simulink model "feedbackLinearizationMambo"  (R2021a)
settings: Solver=VariableStepAuto  StartTime=0.0  StopTime=10  FixedStep=4e-3  RelTol=1e-12
InitFcn:
  | init
values from neighbouring files (symbols this model uses):
  a = 4.7200e-08*13840.8    (= 0.00065328576)    [init.m]
  c = 1.1393e-10*13840.8    (= 1.576882344e-06)    [init.m]
  g = 9.31    [init.m]
  isMambo = true    [init.m]
  J = [Jx;Jy;Jz]    [init.m]
  Jx = 5.82857e-5    (= 5.82857e-05)    [init.m]
  Jy = 7.169148e-5    (= 7.169148e-05)    [init.m]
  Jz = 1e-4    (= 0.0001)    [init.m]
  Ki = [0.1 0.6 0.1]*0    [init.m]
  Kp = [0.6 0.7 1]*50    [init.m]
  Kw = [0.08 0.1 0.2]*100    [init.m]
  l = 0.0624*2    (= 0.1248)    [init.m]
  m = 0.063    [init.m]
  posNED = [57 95 -0.046]    [init.m]
  sigma = [l*a/Jx l*a/Jy l*a/Jz a/m]    [init.m]
  T = 0.0050    (= 0.005)    [init.m]
undefined symbols (not defined in the file or in its folder): DiscIntNeverNeededParam, Earth, init, rho, Vehicle, WGS84
libraries: pid_lib x14, sharedtransform x6, simulink x2, shared6dof x1, aerolibasang x1, aerolibtransform2 x1, vrlib x1
(part 2 of 2)

== system feedbackLinearizationMambo/Controller2/PD Mambo ==
  e : Inport
  Demux : Demux
  Discrete PID Controller : pid_lib/PID Controller  Controller=PD  Form=Parallel  TimeDomain=Discrete-time  UseExternalTs=off  SampleTime=T  IntegratorMethod=Forward Euler  FilterMethod=Forward Euler  ControllerParametersSource=internal  P=0.625617124169113  I=Ki  D=7.14769061437549  UseFilter=on  N=296.310341187165  TunerSelectOption=Transfer Function Based (PID Tuner App)  InitialConditionSource=internal  InitialConditionForIntegrator=0  InitialConditionForFilter=0  DifferentiatorICPrevScaledInput=0  ExternalReset=none  TrackingMode=off  Kt=1  LimitOutput=off  SatLimitsSource=internal  UpperSaturationLimit=inf  LowerSaturationLimit=-inf  LinearizeAsGain=off  AntiWindupMode=none  Kb=1  POutMin=[]  POutMax=[]  IOutMin=[]  IOutMax=[]  DOutMin=[]  DOutMax=[]  NOutMin=[]  NOutMax=[]  SumOutMin=[]  SumOutMax=[]  SaturationOutMin=[]  SaturationOutMax=[]  PParamMin=[]  PParamMax=[]  IParamMin=[]  IParamMax=[]  DParamMin=[]  DParamMax=[]  NParamMin=[]  NParamMax=[]  KbParamMin=[]  KbParamMax=[]  KtParamMin=[]  KtParamMax=[]  KbOutMin=[]  KbOutMax=[]  KtOutMin=[]  KtOutMax=[]  IntegratorOutMin=[]  IntegratorOutMax=[]  FilterOutMin=[]  FilterOutMax=[]  SumI1OutMin=[]  SumI1OutMax=[]  SumI2OutMin=[]  SumI2OutMax=[]  SumI3OutMin=[]  SumI3OutMax=[]  SumI4OutMin=[]  SumI4OutMax=[]  SumDOutMin=[]  SumDOutMax=[]  DifferentiatorOutMin=[]  DifferentiatorOutMax=[]  FilterDiffOutCoefMin=[]  FilterDiffOutCoefMax=[]  ReciprocalOutMin=[]  ReciprocalOutMax=[]  SumDenOutMin=[]  SumDenOutMax=[]  SumNumOutMin=[]  SumNumOutMax=[]  DivideOutMin=[]  DivideOutMax=[]  UdiffTsProdOutMin=[]  UdiffTsProdOutMax=[]  NTsProdOutMin=[]  NTsProdOutMax=[]  UintegralTsProdOutMin=[]  UintegralTsProdOutMax=[]  UngainTsProdOutMin=[]  UngainTsProdOutMax=[]  IntegratorContinuousStateAttributes=''  IntegratorStateMustResolveToSignalObject=off  IntegratorRTWStateStorageClass=Auto  FilterContinuousStateAttributes=''  FilterStateMustResolveToSignalObject=off  FilterRTWStateStorageClass=Auto  ParallelPVariant=InternalParameters  IdealPVariant=Disabled  IVariant=Disabled  DVariant=InternalParameters  IntegratorVariant=Disabled  SatVariant=Disabled  AWVariant=Disabled  PCopyVariant=Disabled  TRVariant=Disabled  FdbkBlocksVariant=Forward  IdealPFdbkVariant=Disabled  SatFdbkVariant=Disabled  DerivativeFilterVariant=ForwardEulerFilter  NVariant=InternalParameters  NCopyVariant=Disabled  FilterICVariant=InternalICsFilter  IntegratorICVariant=Disabled  ExternalResetVariant=Disabled  TRSumVariant=Passthrough  SumFdbkVariant=Disabled  SumVariant=Sum_PD  TsampFilterVariant=InternalTs  TsampNgainVariant=Passthrough  TsampIntegralVariant=Disabled_SignalSpec  ExternalSaturationOutDataTypeStr=Inherit: Same as second input
  Discrete PID Controller1 : pid_lib/PID Controller  Controller=PD  Form=Parallel  TimeDomain=Discrete-time  UseExternalTs=off  SampleTime=T  IntegratorMethod=Forward Euler  FilterMethod=Forward Euler  ControllerParametersSource=internal  P=0.769509803348267  I=Ki  D=8.79166791728825  UseFilter=on  N=296.310341187165  TunerSelectOption=Transfer Function Based (PID Tuner App)  InitialConditionSource=internal  InitialConditionForIntegrator=0  InitialConditionForFilter=0  DifferentiatorICPrevScaledInput=0  ExternalReset=none  TrackingMode=off  Kt=1  LimitOutput=off  SatLimitsSource=internal  UpperSaturationLimit=inf  LowerSaturationLimit=-inf  LinearizeAsGain=off  AntiWindupMode=none  Kb=1  POutMin=[]  POutMax=[]  IOutMin=[]  IOutMax=[]  DOutMin=[]  DOutMax=[]  NOutMin=[]  NOutMax=[]  SumOutMin=[]  SumOutMax=[]  SaturationOutMin=[]  SaturationOutMax=[]  PParamMin=[]  PParamMax=[]  IParamMin=[]  IParamMax=[]  DParamMin=[]  DParamMax=[]  NParamMin=[]  NParamMax=[]  KbParamMin=[]  KbParamMax=[]  KtParamMin=[]  KtParamMax=[]  KbOutMin=[]  KbOutMax=[]  KtOutMin=[]  KtOutMax=[]  IntegratorOutMin=[]  IntegratorOutMax=[]  FilterOutMin=[]  FilterOutMax=[]  SumI1OutMin=[]  SumI1OutMax=[]  SumI2OutMin=[]  SumI2OutMax=[]  SumI3OutMin=[]  SumI3OutMax=[]  SumI4OutMin=[]  SumI4OutMax=[]  SumDOutMin=[]  SumDOutMax=[]  DifferentiatorOutMin=[]  DifferentiatorOutMax=[]  FilterDiffOutCoefMin=[]  FilterDiffOutCoefMax=[]  ReciprocalOutMin=[]  ReciprocalOutMax=[]  SumDenOutMin=[]  SumDenOutMax=[]  SumNumOutMin=[]  SumNumOutMax=[]  DivideOutMin=[]  DivideOutMax=[]  UdiffTsProdOutMin=[]  UdiffTsProdOutMax=[]  NTsProdOutMin=[]  NTsProdOutMax=[]  UintegralTsProdOutMin=[]  UintegralTsProdOutMax=[]  UngainTsProdOutMin=[]  UngainTsProdOutMax=[]  IntegratorContinuousStateAttributes=''  IntegratorStateMustResolveToSignalObject=off  IntegratorRTWStateStorageClass=Auto  FilterContinuousStateAttributes=''  FilterStateMustResolveToSignalObject=off  FilterRTWStateStorageClass=Auto  ParallelPVariant=InternalParameters  IdealPVariant=Disabled  IVariant=Disabled  DVariant=InternalParameters  IntegratorVariant=Disabled  SatVariant=Disabled  AWVariant=Disabled  PCopyVariant=Disabled  TRVariant=Disabled  FdbkBlocksVariant=Forward  IdealPFdbkVariant=Disabled  SatFdbkVariant=Disabled  DerivativeFilterVariant=ForwardEulerFilter  NVariant=InternalParameters  NCopyVariant=Disabled  FilterICVariant=InternalICsFilter  IntegratorICVariant=Disabled  ExternalResetVariant=Disabled  TRSumVariant=Passthrough  SumFdbkVariant=Disabled  SumVariant=Sum_PD  TsampFilterVariant=InternalTs  TsampNgainVariant=Passthrough  TsampIntegralVariant=Disabled_SignalSpec  ExternalSaturationOutDataTypeStr=Inherit: Same as second input
  Discrete PID Controller2 : pid_lib/PID Controller  Controller=PD  Form=Parallel  TimeDomain=Discrete-time  UseExternalTs=off  SampleTime=T  IntegratorMethod=Forward Euler  FilterMethod=Forward Euler  ControllerParametersSource=internal  P=130.980048513602  I=Ki  D=195.85931761802  UseFilter=on  N=189.861187655288  TunerSelectOption=Transfer Function Based (PID Tuner App)  InitialConditionSource=internal  InitialConditionForIntegrator=0  InitialConditionForFilter=0  DifferentiatorICPrevScaledInput=0  ExternalReset=none  TrackingMode=off  Kt=1  LimitOutput=off  SatLimitsSource=internal  UpperSaturationLimit=inf  LowerSaturationLimit=-inf  LinearizeAsGain=off  AntiWindupMode=none  Kb=1  POutMin=[]  POutMax=[]  IOutMin=[]  IOutMax=[]  DOutMin=[]  DOutMax=[]  NOutMin=[]  NOutMax=[]  SumOutMin=[]  SumOutMax=[]  SaturationOutMin=[]  SaturationOutMax=[]  PParamMin=[]  PParamMax=[]  IParamMin=[]  IParamMax=[]  DParamMin=[]  DParamMax=[]  NParamMin=[]  NParamMax=[]  KbParamMin=[]  KbParamMax=[]  KtParamMin=[]  KtParamMax=[]  KbOutMin=[]  KbOutMax=[]  KtOutMin=[]  KtOutMax=[]  IntegratorOutMin=[]  IntegratorOutMax=[]  FilterOutMin=[]  FilterOutMax=[]  SumI1OutMin=[]  SumI1OutMax=[]  SumI2OutMin=[]  SumI2OutMax=[]  SumI3OutMin=[]  SumI3OutMax=[]  SumI4OutMin=[]  SumI4OutMax=[]  SumDOutMin=[]  SumDOutMax=[]  DifferentiatorOutMin=[]  DifferentiatorOutMax=[]  FilterDiffOutCoefMin=[]  FilterDiffOutCoefMax=[]  ReciprocalOutMin=[]  ReciprocalOutMax=[]  SumDenOutMin=[]  SumDenOutMax=[]  SumNumOutMin=[]  SumNumOutMax=[]  DivideOutMin=[]  DivideOutMax=[]  UdiffTsProdOutMin=[]  UdiffTsProdOutMax=[]  NTsProdOutMin=[]  NTsProdOutMax=[]  UintegralTsProdOutMin=[]  UintegralTsProdOutMax=[]  UngainTsProdOutMin=[]  UngainTsProdOutMax=[]  IntegratorContinuousStateAttributes=''  IntegratorStateMustResolveToSignalObject=off  IntegratorRTWStateStorageClass=Auto  FilterContinuousStateAttributes=''  FilterStateMustResolveToSignalObject=off  FilterRTWStateStorageClass=Auto  ParallelPVariant=InternalParameters  IdealPVariant=Disabled  IVariant=Disabled  DVariant=InternalParameters  IntegratorVariant=Disabled  SatVariant=Disabled  AWVariant=Disabled  PCopyVariant=Disabled  TRVariant=Disabled  FdbkBlocksVariant=Forward  IdealPFdbkVariant=Disabled  SatFdbkVariant=Disabled  DerivativeFilterVariant=ForwardEulerFilter  NVariant=InternalParameters  NCopyVariant=Disabled  FilterICVariant=InternalICsFilter  IntegratorICVariant=Disabled  ExternalResetVariant=Disabled  TRSumVariant=Passthrough  SumFdbkVariant=Disabled  SumVariant=Sum_PD  TsampFilterVariant=InternalTs  TsampNgainVariant=Passthrough  TsampIntegralVariant=Disabled_SignalSpec  ExternalSaturationOutDataTypeStr=Inherit: Same as second input
  Discrete PID Controller3 : pid_lib/PID Controller  Controller=PD  Form=Parallel  TimeDomain=Discrete-time  UseExternalTs=off  SampleTime=T  IntegratorMethod=Forward Euler  FilterMethod=Forward Euler  ControllerParametersSource=internal  P=0.0348354109151771  I=Ki  D=1.99510127130573  UseFilter=on  N=145.233498095858  TunerSelectOption=Transfer Function Based (PID Tuner App)  InitialConditionSource=internal  InitialConditionForIntegrator=0  InitialConditionForFilter=0  DifferentiatorICPrevScaledInput=0  ExternalReset=none  TrackingMode=off  Kt=1  LimitOutput=off  SatLimitsSource=internal  UpperSaturationLimit=inf  LowerSaturationLimit=-inf  LinearizeAsGain=off  AntiWindupMode=none  Kb=1  POutMin=[]  POutMax=[]  IOutMin=[]  IOutMax=[]  DOutMin=[]  DOutMax=[]  NOutMin=[]  NOutMax=[]  SumOutMin=[]  SumOutMax=[]  SaturationOutMin=[]  SaturationOutMax=[]  PParamMin=[]  PParamMax=[]  IParamMin=[]  IParamMax=[]  DParamMin=[]  DParamMax=[]  NParamMin=[]  NParamMax=[]  KbParamMin=[]  KbParamMax=[]  KtParamMin=[]  KtParamMax=[]  KbOutMin=[]  KbOutMax=[]  KtOutMin=[]  KtOutMax=[]  IntegratorOutMin=[]  IntegratorOutMax=[]  FilterOutMin=[]  FilterOutMax=[]  SumI1OutMin=[]  SumI1OutMax=[]  SumI2OutMin=[]  SumI2OutMax=[]  SumI3OutMin=[]  SumI3OutMax=[]  SumI4OutMin=[]  SumI4OutMax=[]  SumDOutMin=[]  SumDOutMax=[]  DifferentiatorOutMin=[]  DifferentiatorOutMax=[]  FilterDiffOutCoefMin=[]  FilterDiffOutCoefMax=[]  ReciprocalOutMin=[]  ReciprocalOutMax=[]  SumDenOutMin=[]  SumDenOutMax=[]  SumNumOutMin=[]  SumNumOutMax=[]  DivideOutMin=[]  DivideOutMax=[]  UdiffTsProdOutMin=[]  UdiffTsProdOutMax=[]  NTsProdOutMin=[]  NTsProdOutMax=[]  UintegralTsProdOutMin=[]  UintegralTsProdOutMax=[]  UngainTsProdOutMin=[]  UngainTsProdOutMax=[]  IntegratorContinuousStateAttributes=''  IntegratorStateMustResolveToSignalObject=off  IntegratorRTWStateStorageClass=Auto  FilterContinuousStateAttributes=''  FilterStateMustResolveToSignalObject=off  FilterRTWStateStorageClass=Auto  ParallelPVariant=InternalParameters  IdealPVariant=Disabled  IVariant=Disabled  DVariant=InternalParameters  IntegratorVariant=Disabled  SatVariant=Disabled  AWVariant=Disabled  PCopyVariant=Disabled  TRVariant=Disabled  FdbkBlocksVariant=Forward  IdealPFdbkVariant=Disabled  SatFdbkVariant=Disabled  DerivativeFilterVariant=ForwardEulerFilter  NVariant=InternalParameters  NCopyVariant=Disabled  FilterICVariant=InternalICsFilter  IntegratorICVariant=Disabled  ExternalResetVariant=Disabled  TRSumVariant=Passthrough  SumFdbkVariant=Disabled  SumVariant=Sum_PD  TsampFilterVariant=InternalTs  TsampNgainVariant=Passthrough  TsampIntegralVariant=Disabled_SignalSpec  ExternalSaturationOutDataTypeStr=Inherit: Same as second input
  Mux : Mux
  w : Outport
  wires:
  e/1 -> Demux/1
  Discrete PID Controller2/1 -> Mux/3
  Demux/1 -> Discrete PID Controller/1
  Demux/3 -> Discrete PID Controller2/1
  Discrete PID Controller1/1 -> Mux/2
  Demux/2 -> Discrete PID Controller1/1
  Discrete PID Controller/1 -> Mux/1
  Mux/1 -> w/1
  Demux/4 -> Discrete PID Controller3/1
  Discrete PID Controller3/1 -> Mux/4

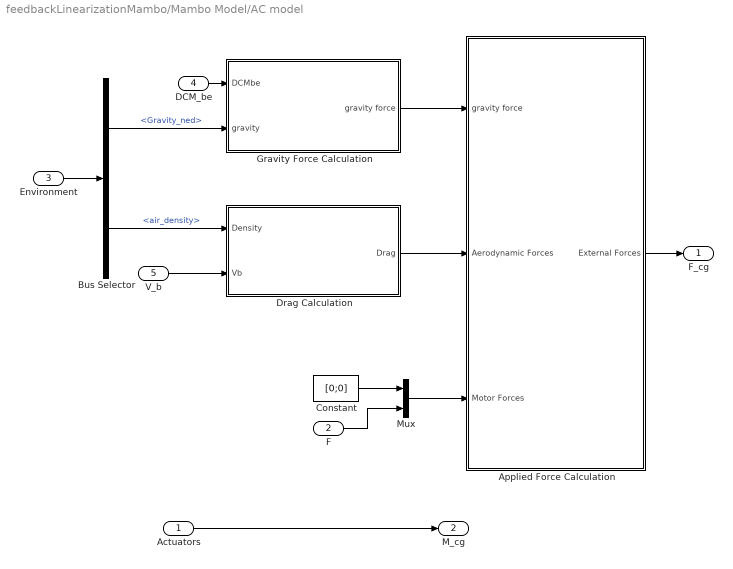
== system feedbackLinearizationMambo/Mambo Model/AC model ==
  Actuators : Inport
  F : Inport  Port=2
  Environment : Inport  Port=3
  DCM_be : Inport  Port=4
  V_b : Inport  Port=5  Unit=m/s
  Applied Force Calculation : Subsystem
  Bus Selector : BusSelector  OutputSignals=Gravity_ned,AtmosphereBus.air_density
  Constant : Constant  Value=[0;0]
  Drag Calculation : Subsystem
  Gravity Force Calculation : Subsystem
  Mux : Mux  Inputs=2
  F_cg : Outport  Unit=N  VectorParamsAs1DForOutWhenUnconnected=off
  M_cg : Outport  Port=2  Unit=N*m  VectorParamsAs1DForOutWhenUnconnected=off
  wires:
  Applied Force Calculation/1(External Forces) -> F_cg/1
  Actuators/1 -> M_cg/1
  Bus Selector/1 -> Gravity Force Calculation/2(gravity)  "<Gravity_ned>"
  Gravity Force Calculation/1(gravity force) -> Applied Force Calculation/1(gravity force)
  Environment/1 -> Bus Selector/1
  Bus Selector/2 -> Drag Calculation/1(Density)  "<air_density>"
  DCM_be/1 -> Gravity Force Calculation/1(DCMbe)
  V_b/1 -> Drag Calculation/2(Vb)
  Drag Calculation/1(Drag) -> Applied Force Calculation/2(Aerodynamic Forces)
  Mux/1 -> Applied Force Calculation/3(Motor Forces)
  Constant/1 -> Mux/1
  F/1 -> Mux/2

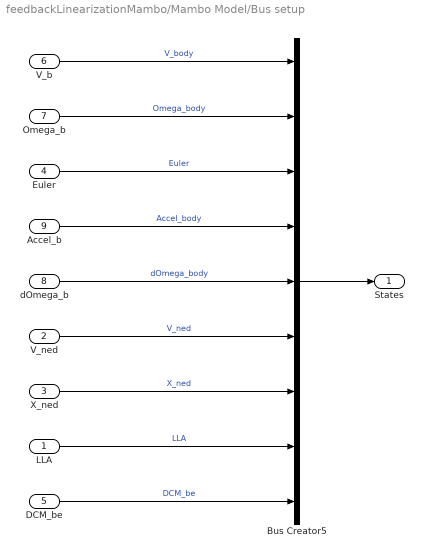
== system feedbackLinearizationMambo/Mambo Model/Bus setup ==
  LLA : Inport  PortDimensions=3
  V_ned : Inport  Port=2  Unit=m/second  PortDimensions=3
  X_ned : Inport  Port=3  Unit=m  PortDimensions=3
  Euler : Inport  Port=4  Unit=rad  PortDimensions=3
  DCM_be : Inport  Port=5  PortDimensions=[3 3]
  V_b : Inport  Port=6  Unit=m/s  PortDimensions=3
  Omega_b : Inport  Port=7  Unit=rad/s  PortDimensions=3
  dOmega_b : Inport  Port=8  Unit=rad/s^2  PortDimensions=3
  Accel_b : Inport  Port=9  Unit=m/s^2  PortDimensions=3
  Bus Creator5 : BusCreator  Inputs=9  OutDataTypeStr=Bus: StatesBus  NonVirtualBus=on
  States : Outport  VectorParamsAs1DForOutWhenUnconnected=off
  wires:
  Bus Creator5/1 -> States/1
  V_b/1 -> Bus Creator5/1  "V_body"
  Omega_b/1 -> Bus Creator5/2  "Omega_body"
  Euler/1 -> Bus Creator5/3  "Euler"
  X_ned/1 -> Bus Creator5/7  "X_ned"
  Accel_b/1 -> Bus Creator5/4  "Accel_body"
  LLA/1 -> Bus Creator5/8  "LLA"
  dOmega_b/1 -> Bus Creator5/5  "dOmega_body"
  DCM_be/1 -> Bus Creator5/9  "DCM_be"
  V_ned/1 -> Bus Creator5/6  "V_ned"

== system feedbackLinearizationMambo/Mambo Model/Position on Earth ==
  Xe : Inport  Unit=m
  Flat Earth to LLA : aerolibtransform2/Flat Earth to LLA  units=Metric (MKS)  ptype=Earth (WGS84)  F=1/298.257223563  R=6378137  refPosPort=off  LL0=init.posLLA(1:2)  psi=Vehicle.PositionOnEarth.FlatEarthToLLA.xAxis
  Mux : Mux  Inputs=2
  href : Constant  Value=Vehicle.PositionOnEarth.href
  LLA : Outport  VectorParamsAs1DForOutWhenUnconnected=off
  wires:
  Mux/1 -> LLA/1
  Xe/1 -> Flat Earth to LLA/1
  Flat Earth to LLA/1 -> Mux/1
  Flat Earth to LLA/2 -> Mux/2
  href/1 -> Flat Earth to LLA/2

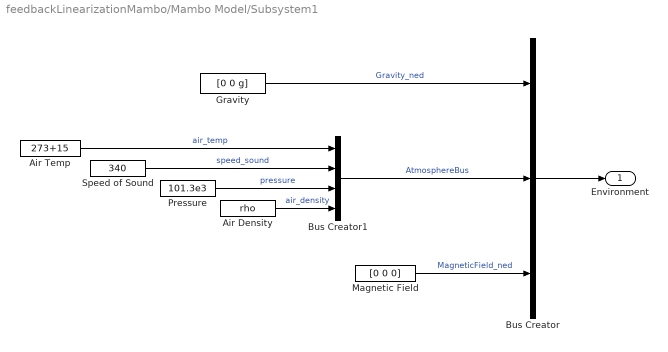
== system feedbackLinearizationMambo/Mambo Model/Subsystem1 ==
  Air Density : Constant  Value=rho
  Air Temp : Constant  Value=273+15
  Bus Creator : BusCreator  Inputs=3  OutDataTypeStr=Bus: EnvironmentBus  NonVirtualBus=on
  Bus Creator1 : BusCreator  Inputs=4  OutDataTypeStr=Bus: AtmosphereBus  NonVirtualBus=on
  Gravity : Constant  Value=[0 0 g]
  Magnetic Field : Constant  Value=[0 0 0]
  Pressure : Constant  Value=101.3e3
  Speed of Sound : Constant  Value=340
  Environment : Outport  VectorParamsAs1DForOutWhenUnconnected=off
  wires:
  Bus Creator1/1 -> Bus Creator/2  "AtmosphereBus"
  Gravity/1 -> Bus Creator/1  "Gravity_ned"
  Air Density/1 -> Bus Creator1/4  "air_density"
  Air Temp/1 -> Bus Creator1/1  "air_temp"
  Speed of Sound/1 -> Bus Creator1/2  "speed_sound"
  Magnetic Field/1 -> Bus Creator/3  "MagneticField_ned"
  Bus Creator/1 -> Environment/1
  Pressure/1 -> Bus Creator1/3  "pressure"

== system feedbackLinearizationMambo/Mambo Model/AC model/Applied Force Calculation ==
  gravity force : Inport  Unit=N
  Aerodynamic Forces : Inport  Port=2  Unit=N
  Motor Forces : Inport  Port=3  Unit=N
  Add1 : Sum  Inputs=+++
  Signal Specification : SignalSpecification  Dimensions=3
  External Forces : Outport  Unit=N  VectorParamsAs1DForOutWhenUnconnected=off
  wires:
  Add1/1 -> Signal Specification/1
  Motor Forces/1 -> Add1/3  "Motor Thrust"
  Aerodynamic Forces/1 -> Add1/2
  gravity force/1 -> Add1/1
  Signal Specification/1 -> External Forces/1

== system feedbackLinearizationMambo/Mambo Model/AC model/Drag Calculation ==
  Density : Inport  Unit=kg/m^3
  Vb : Inport  Port=2  Unit=m/second
  Drag Calc : Subsystem
  Gain3 : Gain  Gain=-1
  Product : Product  RndMeth=Zero
  Sign : Signum  ZeroCross=off
  Drag : Outport  Unit=N  VectorParamsAs1DForOutWhenUnconnected=off
  wires:
  Density/1 -> Drag Calc/1(Density)
  Sign/1 -> Gain3/1
  Drag Calc/1(drag) -> Product/1
  Gain3/1 -> Product/2
  Product/1 -> Drag/1  "xDrag"
  Vb/1 -> Sign/1, Drag Calc/2(vel)

== system feedbackLinearizationMambo/Mambo Model/AC model/Gravity Force Calculation ==
  DCMbe : Inport
  gravity : Inport  Port=2  Unit=m/s^2
  Gain1 : Gain  Gain=Vehicle.Airframe.mass
  Product : Product  Multiplication=Matrix(*)
  gravity force : Outport  Unit=N  VectorParamsAs1DForOutWhenUnconnected=off
  wires:
  gravity/1 -> Gain1/1
  Gain1/1 -> Product/2  "gravity force NED"
  Product/1 -> gravity force/1
  DCMbe/1 -> Product/1

== system feedbackLinearizationMambo/Mambo Model/AC model/Drag Calculation/Drag Calc ==
  Density : Inport  Unit=kg/m^3
  vel : Inport  Port=2  Unit=m/s
  Dynamic Pressure : aerolibasang/Dynamic Pressure
  Gain : Gain  Gain=[.25 .25]
  Mux1 : Mux  Inputs=2
  Product : Product  Inputs=3  RndMeth=Zero
  diameter : Constant  Value=Vehicle.Airframe.diameter  SampleTime=0
  dragCoeff : Constant  Value=Vehicle.Airframe.Cdx  SampleTime=0
  drag : Outport  Unit=N  VectorParamsAs1DForOutWhenUnconnected=off
  wires:
  Product/1 -> drag/1
  dragCoeff/1 -> Product/3  "Cd"
  Dynamic Pressure/1 -> Product/1  "q"
  diameter/1 -> Gain/1, Mux1/2
  Mux1/1 -> Product/2  "S"
  Gain/1 -> Mux1/1
  vel/1 -> Dynamic Pressure/1
  Density/1 -> Dynamic Pressure/2

== matlab function feedbackLinearizationMambo/w2Toques2/MATLAB Function ==
  data: m input; delta output; n input; o input; k input
function delta = const2delta(m,n,o,k)
 d1 = (k-2*n+o)/4;
 d2 = (k+2*m-o)/4;
 d3 = (k+2*n+o)/4;
 d4 = (k-2*m-o)/4;
 
 delta = [d1;d2;d3;d4];

== matlab function feedbackLinearizationMambo/w2Toques2/MATLAB Function1 ==
  data: delta input; w2 output
function w2 = delta2w2(delta)
    aux = delta.*13840.8;
    w = abs(aux).^0.5;
    w2 = w.^2.*sign(delta);

== matlab function feedbackLinearizationMambo/w2Toques2/MATLAB Function2 ==
  data: w2 input; tauPhi output; tauTheta output; tauPsi output; F output
function [tauPhi,tauTheta,tauPsi,F] = w2toque(w2)
    tauPhi = (0.0624*2)*4.7200e-08*(w2(2)-w2(4));
    tauTheta = (0.0624*2)*4.7200e-08*(w2(3)-w2(1));
    tauPsi = 1.1393e-10*(w2(3)+w2(1)-w2(2)-w2(4));
    F = 4.7200e-08*(w2(3)+w2(1)+w2(2)+w2(4));

== matlab function feedbackLinearizationMambo/ 1 ==
  data: quart input; e input; w input size=4; m output; v input; n output; o output; sigma parameter; linearVel input; J parameter; k output; g parameter
function [m, n, o, k] = feedbackLin(quart,e, w, v, sigma,linearVel, J,g)

ml = w(1);
nl = w(2);
ol = w(3);
kl = w(4);

q0 = quart(1);
q1 = quart(2);
q2 = quart(3);
q3 = quart(4);

p = v(1);
q = v(2);
r = v(3);

Jx = J(1);
Jy = J(2);
Jz = J(3);

vy = linearVel(2);
vx = linearVel(1);

A = [ q0 + q1^2/q0,  q3 + q1*q2/q0,  -q2 + q1*q3/q0;
      -q3 + q1*q2/q0,  q0 + q2^2/q0,   q1 + q2*q3/q0;
      q2 + q1*q3/q0,  -q1 + q2*q3/q0,  q0 + q3^2/q0];
  
dq0 = 1/2*(-q1*p - q2*q - q3*r);
dq1 = 1/2*(q0*p - q3*q + q2*r);
dq2 = 1/2*(q3*p + q0*q - q1*r);
dq3 = 1/2*(-q2*p + q1*q + q0*r);

dp = (Jy-Jz)/Jx*q*r;
dq = (Jz-Jx)/Jy*p*r;
dr = (Jx-Jy)/Jz*q*p;

SigmaQ1 = sigma(1);
SigmaQ2 = sigma(2);
SigmaQ3 = sigma(3);
SigmaZ = sigma(4);

B = [(2*ml - (dq0*p - dq3*q + dq2*r) - (q0*dp-q3*dq+q2*dr))/SigmaQ1;
     (2*nl - (dq3*p + dq0*q - dq1*r) - (q3*dp+q0*dq-q1*dr))/SigmaQ2;
     (2*ol - (-dq2*p + dq3*q + dq0*r) - (-q2*dp+q1*dq+q0*dr))/SigmaQ3];
 
C = A*B;

phi = e(1);
theta = e(2);

m = C(1);
n = C(2);
o = C(3);
k = (kl-(q*vx-p*vy+g*cos(phi)*cos(theta)))/SigmaZ;

== matlab function feedbackLinearizationMambo/ 2 ==
  data: quart input; e input; w input size=4; m output; v input; n output; o output; sigma parameter; linearVel input; J parameter; k output; g parameter
function [m, n, o, k] = feedbackLin(quart,e, w, v, sigma,linearVel, J,g)

ml = w(1);
nl = w(2);
ol = w(3);
kl = w(4);

q0 = quart(1);
q1 = quart(2);
q2 = quart(3);
q3 = quart(4);

p = v(1);
q = v(2);
r = v(3);

Jx = J(1);
Jy = J(2);
Jz = J(3);

vy = linearVel(2);
vx = linearVel(1);

A = [ q0 + q1^2/q0,  q3 + q1*q2/q0,  -q2 + q1*q3/q0;
      -q3 + q1*q2/q0,  q0 + q2^2/q0,   q1 + q2*q3/q0;
      q2 + q1*q3/q0,  -q1 + q2*q3/q0,  q0 + q3^2/q0];
  
dq0 = 1/2*(-q1*p - q2*q - q3*r);
dq1 = 1/2*(q0*p - q3*q + q2*r);
dq2 = 1/2*(q3*p + q0*q - q1*r);
dq3 = 1/2*(-q2*p + q1*q + q0*r);

dp = (Jy-Jz)/Jx*q*r;
dq = (Jz-Jx)/Jy*p*r;
dr = (Jx-Jy)/Jz*q*p;

SigmaQ1 = sigma(1);
SigmaQ2 = sigma(2);
SigmaQ3 = sigma(3);
SigmaZ = sigma(4);

B = [(2*ml - (dq0*p - dq3*q + dq2*r) - (q0*dp-q3*dq+q2*dr))/SigmaQ1;
     (2*nl - (dq3*p + dq0*q - dq1*r) - (q3*dp+q0*dq-q1*dr))/SigmaQ2;
     (2*ol - (-dq2*p + dq3*q + dq0*r) - (-q2*dp+q1*dq+q0*dr))/SigmaQ3];
 
C = A*B;

phi = e(1);
theta = e(2);

m = C(1);
n = C(2);
o = C(3);
k = (kl-(q*vx-p*vy+g*cos(phi)*cos(theta)))/SigmaZ;

== matlab function feedbackLinearizationMambo/w2Toques1/MATLAB Function ==
  data: m input; delta output; n input; o input; k input
function delta = const2delta(m,n,o,k)
 d1 = (k-2*n+o)/4;
 d2 = (k+2*m-o)/4;
 d3 = (k+2*n+o)/4;
 d4 = (k-2*m-o)/4;
 
 delta = [d1;d2;d3;d4];

== matlab function feedbackLinearizationMambo/Non Linear Model/MATLAB Function1 ==
  data: F input; force output; m input; g input; euler input
function force = intertial2body(F,m,g,euler)
%         force = m*g*[sin(euler(2));
%                      cos(euler(2))*sin(euler(1));
%                      cos(euler(2))*cos(euler(1))];
                 
    phi = euler(1);
    theta = euler(2);
    psi = euler(3);
    Rz = [cos(psi) -sin(psi) 0; 
        sin(psi) cos(psi) 0;
        0 0 1];
    Ry = [cos(theta) 0 sin(theta); 
        0 1 0; 
        -sin(theta) 0 cos(theta)];
    Rx = [1 0 0;
        0 cos(phi) -sin(phi);
        0 sin(phi) cos(phi)];
    R = Rz*Ry*Rx;
    P = inv(R)*[0;0;m*g];
    force=P+[0;0;F];

== matlab function feedbackLinearizationMambo/Non Linear Model/MATLAB Function2 ==
  data: vBody input; vInertial output; euler input
function vInertial = body2Inertial(vBody,euler)
    phi = euler(1);
    theta = euler(2);
    psi = euler(3);
    Rz = [cos(psi) -sin(psi) 0; 
        sin(psi) cos(psi) 0;
        0 0 1];
    Ry = [cos(theta) 0 sin(theta); 
        0 1 0; 
        -sin(theta) 0 cos(theta)];
    Rx = [1 0 0;
        0 cos(phi) -sin(phi);
        0 sin(phi) cos(phi)];
    R = Rz*Ry*Rx;
    vInertial = R*vBody;

== matlab function feedbackLinearizationMambo/w2Toques1/MATLAB Function1 ==
  data: delta input; w2 output
function w2 = delta2w2(delta)
    aux = delta.*13840.8;
    w = abs(aux).^0.5;
    w2 = w.^2.*sign(delta);

== matlab function feedbackLinearizationMambo/w2Toques1/MATLAB Function2 ==
  data: w2 input; tauPhi output; tauTheta output; tauPsi output; F output
function [tauPhi,tauTheta,tauPsi,F] = w2toque(w2)
    tauPhi = (0.0624*2)*4.7200e-08*(w2(2)-w2(4));
    tauTheta = (0.0624*2)*4.7200e-08*(w2(3)-w2(1));
    tauPsi = 1.1393e-10*(w2(3)+w2(1)-w2(2)-w2(4));
    F = 4.7200e-08*(w2(3)+w2(1)+w2(2)+w2(4));
